simulink model "SysTestModel"  (R2025b)
settings: Solver=VariableStepAuto  StartTime=0.0  StopTime=SimTime  RelTol=1e-3
values from neighbouring files (symbols this model uses):
  A = [0.92  0.08  0.00 ... (first row only)    [SysTest.m]
  B = [0.10  0.00 ... (first row only)    [SysTest.m]
  C = [1 0 0 ... (first row only)    [SysTest.m]
  D = zeros(2,2)    [SysTest.m]
  P = diag([5, 5])    [SysTest.m]
  R = diag([0.05, 0.05])    [SysTest.m]
  x0 = [0; 0; 0]    [SysTest.m]
libraries: Algebraic_MPC x1
settings Model: Creator=Talha  LastModifiedBy=Talha
settings OptimizationCC: ReuseModelBlockBuffer=off
settings RTWCC: GPUComputeCapability=3.5

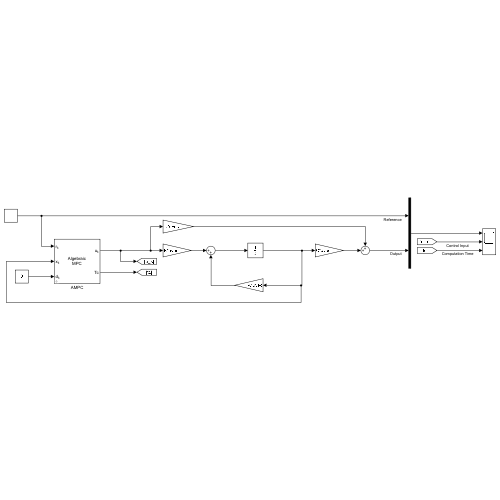
[thumbnail: Simulink's stored preview of the top-level diagram]
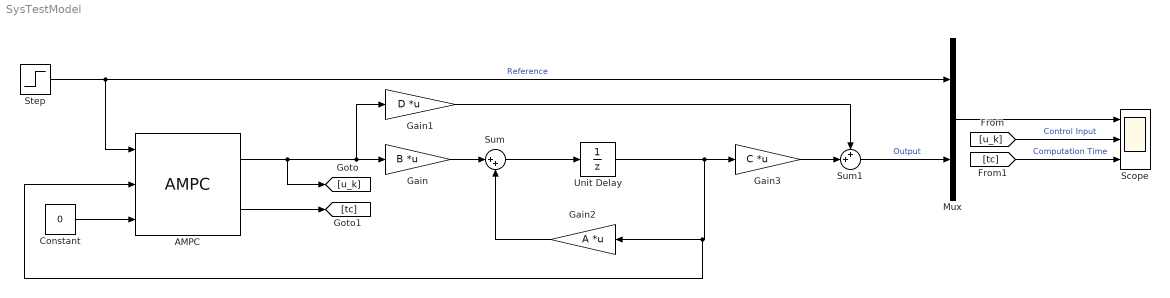
== system SysTestModel ==
  AMPC : Algebraic_MPC/AMPC  System_Model=plant  x0=x0  E=E  F=F  Rate_enable=off  Integral_Enable=off  Disturbance_Enable=off  u_min=u_min  u_max=u_max  u_dot_max=du_max  FB_Cons=off  y_min=y_min  y_max=y_max  Q=Q  P=P  R=R  N_State=N  Parameter17=off
      settings: SourceProductName=Algebraic MPC
  Constant : Constant  Value=0
  Gain : Gain  Gain=B  Multiplication=Matrix(K*u) (u vector)
  Gain1 : Gain  Gain=D  Multiplication=Matrix(K*u) (u vector)
  Gain2 : Gain  Gain=A  Multiplication=Matrix(K*u) (u vector)
  Gain3 : Gain  Gain=C  Multiplication=Matrix(K*u) (u vector)
  Mux : Mux  Inputs=2
  Scope : Scope  NumInputPorts=3
      settings: SampleTime=Ts  ActiveDisplayYMinimum=-0.25687239642049792  ActiveDisplayYMaximum=2.3118515677844815
  Step : Step  After=2  SampleTime=0
  Sum : Sum  Inputs=|++
  Sum1 : Sum  Inputs=++|
  Unit Delay : UnitDelay  InitialCondition=x0  SampleTime=-1  HasFrameUpgradeWarning=on
  wires:
  Constant/1 -> AMPC/3
  Step/1 -> AMPC/1, Mux/1  "Reference"
  AMPC/1 -> [u_k], Gain1/1, Gain/1
  AMPC/2 -> [tc]
  Gain/1 -> Sum/1
  Gain2/1 -> Sum/2
  Sum/1 -> Unit Delay/1
  Gain1/1 -> Sum1/1
  Unit Delay/1 -> Gain3/1, AMPC/2, Gain2/1
  Gain3/1 -> Sum1/2
  Sum1/1 -> Mux/2  "Output"
  Mux/1 -> Scope/1
  [u_k] -> Scope/2  "Control Input"
  [tc] -> Scope/3  "Computation Time"
